simulink model "adaptive_mrac"  (R2020a)
settings: Solver=FixedStepAuto  StartTime=0.0  StopTime=89.99  FixedStep=0.01  RelTol=1e-3
values from neighbouring files (symbols this model uses):
  gamma_r = 0.03    [cases_test.m]    (also in cases_tests_lr.m = gamma_r_0 * i; mrac_model_const_ref.m = params(6); mrac_model_lr.m = params(5); mrac_model_lr_init.m = params(8))
  gamma_x = [0.5; 0.5]    [cases_test.m]    (also in cases_tests_lr.m = gamma_x_0 * i; mrac_model_const_ref.m = params(4:5); mrac_model_e2y.m = params(5:6); mrac_model_e2y_2delay.m = params(7:8))
  k_r0 = k_r0_list(:, plant_case)    [cases_test.m]    (also in mrac_model_const_ref.m = params(3); mrac_model_lr_init.m = params(3); mrac_model_lr_init_low_pass.m = params(3); mrac_pursuit.m = params(3))
  k_x0 = k_x0_list(:, plant_case)    [cases_test.m]    (also in mrac_model_const_ref.m = [-params(1); params(2)]; mrac_model_e2y.m = params(1:2); mrac_model_e2y_2delay.m = params(1:2); mrac_model_lr_init.m = [-params(1); params(2)])
  ref_sys = canon(ref_sys, 'modal')    [cases_test.m]    (also in cases_tests_lr.m; mrac_model.m = ss([tf_cl_pade; s*tf_cl_pade]); mrac_model_e2y.m = ss([tf_cl_pade; s*tf_cl_pade]); mrac_model_e2y_2delay.m = ss([tf_cl_pade; s*tf_cl_pade]))
undefined symbols (not defined in the file or in its folder): case_, ref_x0
settings Model: OrderedModelArguments=off  Creator=lorenzoterenzi  LastModifiedBy=lorenzoterenzi

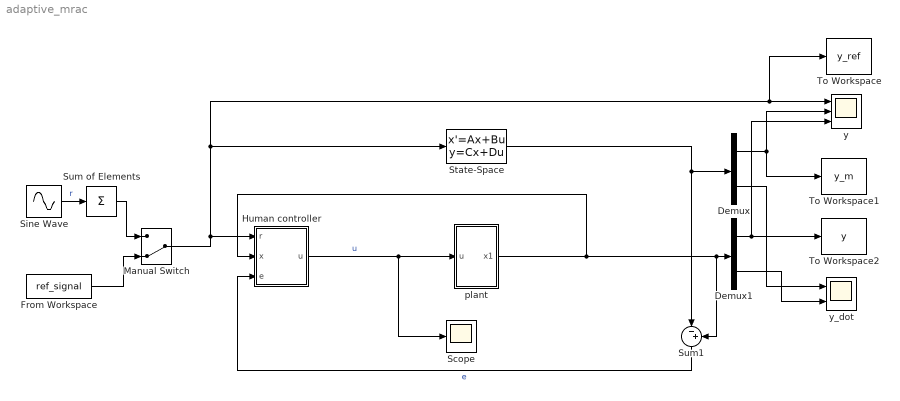
== system adaptive_mrac ==
  Demux : Demux  Outputs=2
  Demux1 : Demux  Outputs=2
  From Workspace : FromWorkspace  VariableName=ref_signal
  Human controller : Subsystem
  Manual Switch : ManualSwitch  CurrentSetting=0
  Scope : Scope
  Sine Wave : Sin  Amplitude=[1.186, 1.121, 0.991, 0.756, 0.447, 0.245, 0.123, 0.061, 0.036, 0.025]  Frequency=[0.23, 0.384, 0.614, 0.997, 1.687, 2.608, 4.065, 6.596, 10.661, 17.564]  Phase=[0.974, -3.02, 0.744, -2.300, 2.984, -2.513, 2.211, 1.0, -2.225, 2.210]  SampleTime=0
  State-Space : StateSpace  A=ref_sys.A  B=ref_sys.B  C=ref_sys.C  D=ref_sys.D  InitialCondition=ref_x0
  Sum of Elements : Sum  Inputs=+
  Sum1 : Sum  Inputs=|-+
  To Workspace : ToWorkspace  VariableName=y_ref  SaveFormat=Timeseries  SampleTime=-1
  To Workspace1 : ToWorkspace  VariableName=y_m  SaveFormat=Timeseries  SampleTime=-1
  To Workspace2 : ToWorkspace  VariableName=y  SaveFormat=Timeseries  SampleTime=-1
  plant : Subsystem
  y : Scope  NumInputPorts=3
  y_dot : Scope  NumInputPorts=2
  wires:
  Demux/2 -> y_dot/1
  Sum1/1 -> Human controller/3(e)  "e"
  Demux1/2 -> y_dot/2
  Demux/1 -> y/2, To Workspace1/1
  Manual Switch/1 -> Human controller/1(r), y/1, To Workspace/1, State-Space/1
  Sine Wave/1 -> Sum of Elements/1  "r"
  Human controller/1(u) -> Scope/1, plant/1(u)  "u"
  State-Space/1 -> Demux/1, Sum1/1
  Demux1/1 -> y/3, To Workspace2/1
  Sum of Elements/1 -> Manual Switch/1
  plant/1(x1) -> Human controller/2(x), Sum1/2, Demux1/1
  From Workspace/1 -> Manual Switch/2

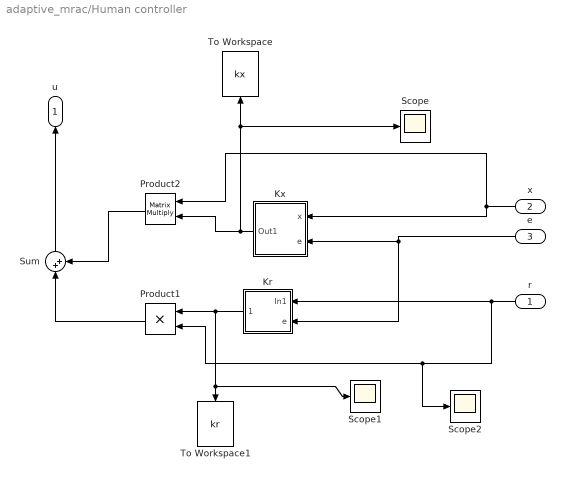
== system adaptive_mrac/Human controller ==
  r : Inport
  x : Inport  Port=2
  e : Inport  Port=3
  Kr : Subsystem
  Kx : Subsystem
  Product1 : Product
  Product2 : Product  Multiplication=Matrix(*)
  Scope : Scope
  Scope1 : Scope
  Scope2 : Scope
  Sum : Sum  Inputs=|++
  To Workspace : ToWorkspace  VariableName=kx  SaveFormat=Timeseries  SampleTime=-1
  To Workspace1 : ToWorkspace  VariableName=kr  SaveFormat=Timeseries  SampleTime=-1
  u : Outport
  wires:
  Kx/1(Out1) -> Product2/2, To Workspace/1, Scope/1
  x/1 -> Product2/1, Kx/1(x)
  r/1 -> Scope2/1, Product1/2, Kr/1(In1)
  Product2/1 -> Sum/2
  Product1/1 -> Sum/1
  e/1 -> Kx/2(e), Kr/2(e)
  Sum/1 -> u/1
  Kr/1(Out1) -> Scope1/1, To Workspace1/1, Product1/1

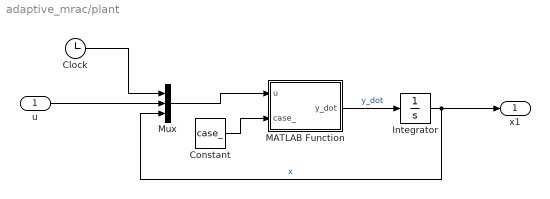
== system adaptive_mrac/plant ==
  u : Inport
  Clock : Clock
  Constant : Constant  Value=case_
  Integrator : Integrator  InitialCondition=[0;0]
  MATLAB Function : MATLAB Function  TreatAsAtomicUnit=on
  Mux : Mux  Inputs=3
  x1 : Outport
  wires:
  Mux/1 -> MATLAB Function/1(u)
  Integrator/1 -> x1/1, Mux/3  "x"
  MATLAB Function/1(y_dot) -> Integrator/1  "y_dot"
  Clock/1 -> Mux/1
  Constant/1 -> MATLAB Function/2(case_)
  u/1 -> Mux/2

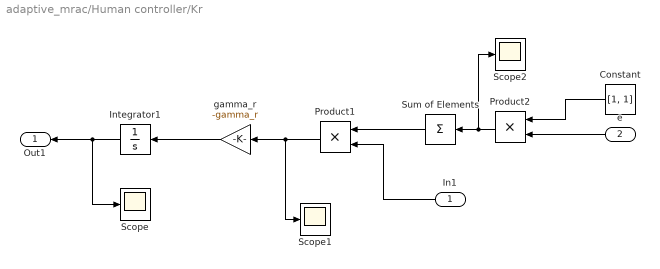
== system adaptive_mrac/Human controller/Kr ==
  In1 : Inport
  e : Inport  Port=2
  Constant : Constant  Value=[1, 1]
  Integrator1 : Integrator  InitialCondition=k_r0
  Product1 : Product
  Product2 : Product
  Scope : Scope
  Scope1 : Scope
  Scope2 : Scope
  Sum of Elements : Sum  Inputs=+
  gamma_r : Gain  Gain=-gamma_r
  Out1 : Outport
  wires:
  In1/1 -> Product1/2
  Product1/1 -> Scope1/1, gamma_r/1
  Product2/1 -> Scope2/1, Sum of Elements/1
  e/1 -> Product2/2
  Sum of Elements/1 -> Product1/1
  Integrator1/1 -> Out1/1, Scope/1
  Constant/1 -> Product2/1
  gamma_r/1 -> Integrator1/1

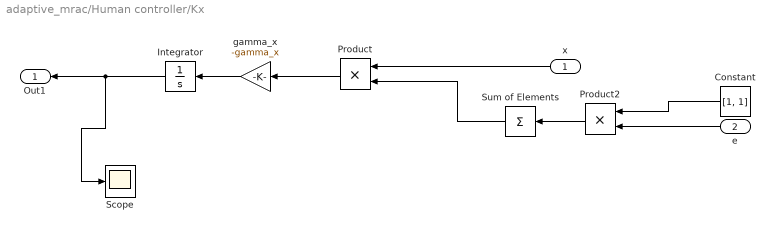
== system adaptive_mrac/Human controller/Kx ==
  x : Inport
  e : Inport  Port=2
  Constant : Constant  Value=[1, 1]
  Integrator : Integrator  InitialCondition=k_x0
  Product : Product
  Product2 : Product
  Scope : Scope
  Sum of Elements : Sum  Inputs=+
  gamma_x : Gain  Gain=-gamma_x
  Out1 : Outport  PortDimensions=[2, 1]
  wires:
  x/1 -> Product/1
  e/1 -> Product2/2
  Product2/1 -> Sum of Elements/1
  Sum of Elements/1 -> Product/2
  Integrator/1 -> Scope/1, Out1/1
  Constant/1 -> Product2/1
  gamma_x/1 -> Integrator/1
  Product/1 -> gamma_x/1

== matlab function adaptive_mrac/plant/MATLAB Function ==
  data: u input size=4; y_dot output size=2; case_ input
function y_dot = fcn(u, case_)
    t = u(1);
    u_c = u(2);
    y_prev = u(3:4);
    y_dot = models.peter_plant(case_, t, u_c, y_prev);
end


% function y_dot = peter_plant(case_, t, u, y_prev)
%     % case 1: first to second order system transition
%     if case_ == 1
%         M = -1;
%         G = -100;
%     % case 2: second to first order transition
%     elseif case_ == 2 
%         M = 91;
%         G = 100;
%     elseif case_ == 3    
%         M = 50;
%         G = 0.5;
%     elseif case_ == 4
%         M = 50;
%         G = 100;
%     else
%         G = 0;
%         M = 0;
%     end
% 
%     omega_b1 = 6;
%     omega_b2 = 0.2;
%     k_c1 = 90;
%     k_c2 = 30;
% 
%     omega_b = omega_b1 + (omega_b2 - omega_b1)./(1 + exp(-G * (t - M)));
%     k_c = k_c1 + (k_c2 - k_c1)./(1 + exp(-G * (t - M)));
% 
%     A = [0, 1; 0, omega_b];
%     B = [0; k_c];
%     y_dot = A*y_prev + B*u;
% end
